simulink model "SigAndParam"  (R2020a)
settings: Solver=VariableStepAuto  StartTime=0.0  StopTime=10.0  RelTol=1e-3
libraries: simulink x1, dspsigops x1
settings Model: Creator=ashok  LastModifiedBy=ashok

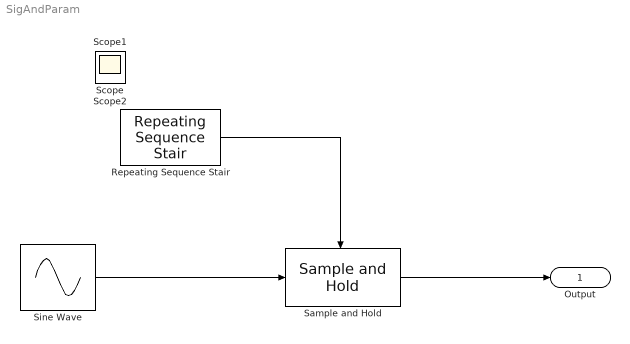
== system SigAndParam ==
  Repeating Sequence Stair : simulink/Sources/Repeating Sequence Stair  OutValues=[1 0].'  tsamp=-1  OutMin=[]  OutMax=[]  OutDataTypeStr=double  OutputDataTypeScalingMode=double  OutDataType=fixdt(0,8)  ConRadixGroup=Best Precision: Vector-wise  OutScaling=2^-12
  Sample and Hold : dspsigops/Sample and Hold  trig=Rising edge  initCond=0  latchinput=off
  Sine Wave : Sin  Amplitude=5  SampleTime=0
  Output : Outport
  Scope : Scope
  Scope1 : Scope
  Scope2 : Scope
  wires:
  Sine Wave/1 -> Sample and Hold/1
  Repeating Sequence Stair/1 -> Sample and Hold/Trigger
  Sample and Hold/1 -> Output/1
